simulink model "FIR_Direct_Form"  (R2012b)
settings: Solver=ode45  StartTime=0.0  StopTime=10.0  RelTol=1e-3
settings Model: Creator=Ahmad  LastModifiedBy=Ahmad

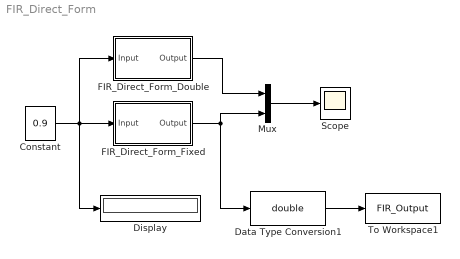
== system FIR_Direct_Form ==
  Constant : Constant  Value=0.9  VectorParams1D=off  OutDataTypeStr=fixdt(1,14,13)  SampleTime=1/50e6
  Data Type Conversion1 : DataTypeConversion  OutDataTypeStr=double
  Display : Display
  FIR_Direct_Form_Double : Subsystem  Tag=FilterWizardSubSystem
      settings: ErrorFcn=dspFilterRealizedInBasicElemsAlgLoopErrFcnCallback
  FIR_Direct_Form_Fixed : Subsystem  Tag=FilterWizardSubSystem
      settings: ErrorFcn=dspFilterRealizedInBasicElemsAlgLoopErrFcnCallback
  Mux : Mux  Inputs=2
  Scope : Scope
      settings: YMin=0.1  YMax=0.85
  To Workspace1 : ToWorkspace  VariableName=FIR_Output  SampleTime=-1  SaveFormat=Timeseries
  wires:
  Constant/1 -> FIR_Direct_Form_Double/1(Input), FIR_Direct_Form_Fixed/1(Input), Display/1
  FIR_Direct_Form_Fixed/1(Output) -> Data Type Conversion1/1, Mux/2
  Data Type Conversion1/1 -> To Workspace1/1
  FIR_Direct_Form_Double/1(Output) -> Mux/1
  Mux/1 -> Scope/1

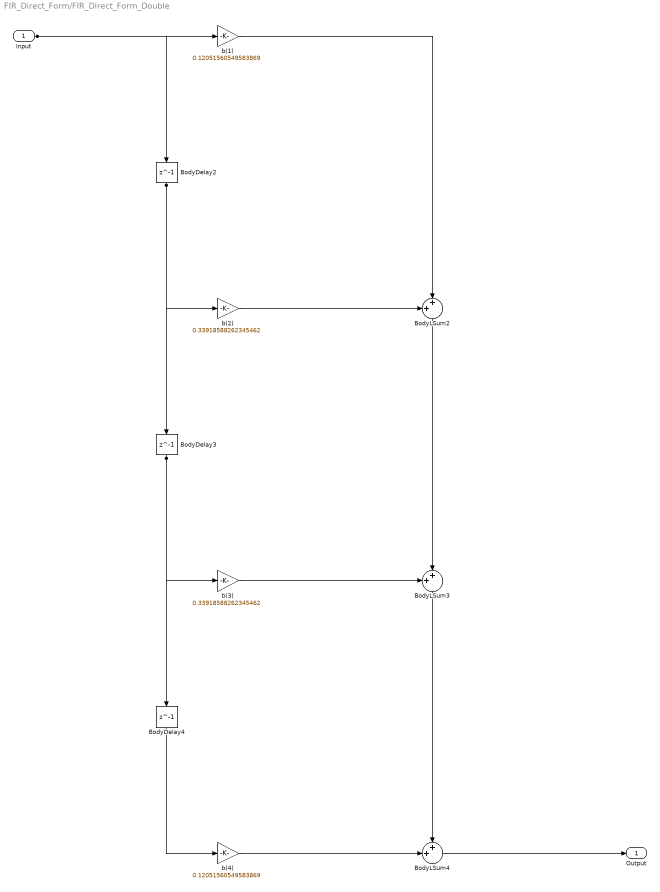
== system FIR_Direct_Form/FIR_Direct_Form_Double ==
  Input : Inport
  BodyDelay2 : Delay  DelayLength=1  InitialCondition=0
  BodyDelay3 : Delay  DelayLength=1  InitialCondition=0
  BodyDelay4 : Delay  DelayLength=1  InitialCondition=0
  BodyLSum2 : Sum  Inputs=++|  RndMeth=Nearest  SaturateOnIntegerOverflow=on  OutDataTypeStr=Inherit: Same as first input
  BodyLSum3 : Sum  Inputs=++|  RndMeth=Nearest  SaturateOnIntegerOverflow=on  OutDataTypeStr=Inherit: Same as first input
  BodyLSum4 : Sum  Inputs=++|  RndMeth=Nearest  SaturateOnIntegerOverflow=on  OutDataTypeStr=Inherit: Same as first input
  b(1) : Gain  Gain=0.12051560549583869  ParamDataTypeStr=double  RndMeth=Nearest  SaturateOnIntegerOverflow=on  OutDataTypeStr=Inherit: Same as input
  b(2) : Gain  Gain=0.33918588262345462  ParamDataTypeStr=double  RndMeth=Nearest  SaturateOnIntegerOverflow=on  OutDataTypeStr=Inherit: Same as input
  b(3) : Gain  Gain=0.33918588262345462  ParamDataTypeStr=double  RndMeth=Nearest  SaturateOnIntegerOverflow=on  OutDataTypeStr=Inherit: Same as input
  b(4) : Gain  Gain=0.12051560549583869  ParamDataTypeStr=double  RndMeth=Nearest  SaturateOnIntegerOverflow=on  OutDataTypeStr=Inherit: Same as input
  Output : Outport
  wires:
  Input/1 -> b(1)/1, BodyDelay2/1
  b(1)/1 -> BodyLSum2/2
  BodyDelay2/1 -> b(2)/1, BodyDelay3/1
  b(2)/1 -> BodyLSum2/1
  BodyLSum2/1 -> BodyLSum3/2
  BodyDelay3/1 -> b(3)/1, BodyDelay4/1
  b(3)/1 -> BodyLSum3/1
  BodyLSum3/1 -> BodyLSum4/1
  BodyDelay4/1 -> b(4)/1
  b(4)/1 -> BodyLSum4/2
  BodyLSum4/1 -> Output/1

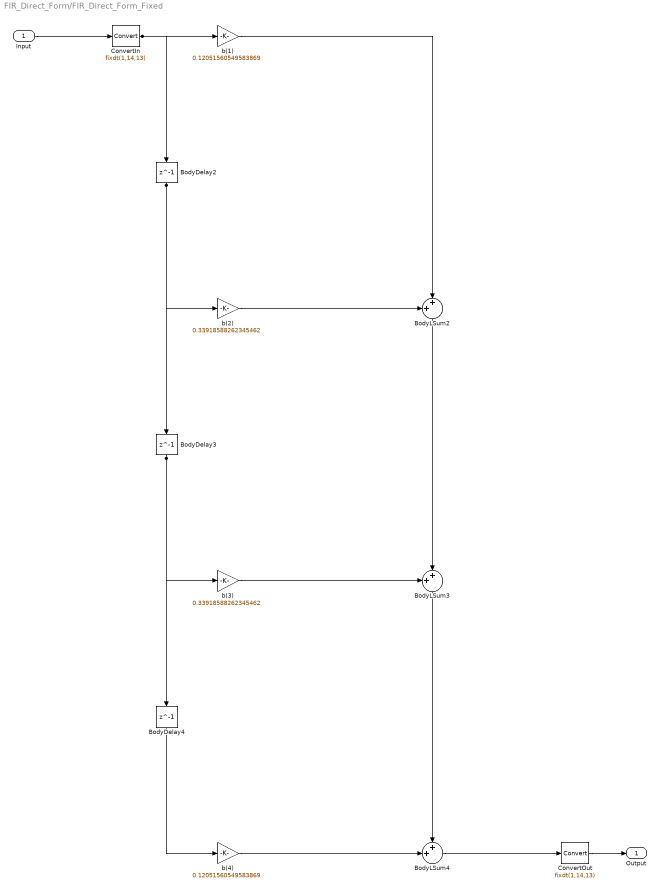
== system FIR_Direct_Form/FIR_Direct_Form_Fixed ==
  Input : Inport
  BodyDelay2 : Delay  DelayLength=1  InitialCondition=0
  BodyDelay3 : Delay  DelayLength=1  InitialCondition=0
  BodyDelay4 : Delay  DelayLength=1  InitialCondition=0
  BodyLSum2 : Sum  Inputs=++|  AccumDataTypeStr=fixdt(1,22,21)  OutDataTypeStr=fixdt(1,24,21)
  BodyLSum3 : Sum  Inputs=++|  AccumDataTypeStr=fixdt(1,22,21)  OutDataTypeStr=fixdt(1,24,21)
  BodyLSum4 : Sum  Inputs=++|  AccumDataTypeStr=fixdt(1,22,21)  OutDataTypeStr=fixdt(1,24,21)
  ConvertIn : DataTypeConversion  OutDataTypeStr=fixdt(1,14,13)  RndMeth=Nearest  SaturateOnIntegerOverflow=on
  ConvertOut : DataTypeConversion  OutDataTypeStr=fixdt(1,14,13)
  b(1) : Gain  Gain=0.12051560549583869  ParamDataTypeStr=fixdt(1,9,8)  OutDataTypeStr=fixdt(1,23,21)
  b(2) : Gain  Gain=0.33918588262345462  ParamDataTypeStr=fixdt(1,9,8)  OutDataTypeStr=fixdt(1,23,21)
  b(3) : Gain  Gain=0.33918588262345462  ParamDataTypeStr=fixdt(1,9,8)  OutDataTypeStr=fixdt(1,23,21)
  b(4) : Gain  Gain=0.12051560549583869  ParamDataTypeStr=fixdt(1,9,8)  OutDataTypeStr=fixdt(1,23,21)
  Output : Outport
  wires:
  Input/1 -> ConvertIn/1
  b(1)/1 -> BodyLSum2/2
  ConvertIn/1 -> b(1)/1, BodyDelay2/1
  BodyDelay2/1 -> b(2)/1, BodyDelay3/1
  b(2)/1 -> BodyLSum2/1
  BodyLSum2/1 -> BodyLSum3/2
  BodyDelay3/1 -> b(3)/1, BodyDelay4/1
  b(3)/1 -> BodyLSum3/1
  BodyLSum3/1 -> BodyLSum4/1
  BodyDelay4/1 -> b(4)/1
  b(4)/1 -> BodyLSum4/2
  BodyLSum4/1 -> ConvertOut/1
  ConvertOut/1 -> Output/1
